simulink model "ZAD2_Model"  (R2018a)
settings: Solver=ode45  StartTime=0.0  StopTime=tend  MaxStep=Tp  RelTol=1e-3
values from neighbouring files (symbols this model uses):
  initConditionsAcc = [0 0]    [ZAD2_Init.m]
  initConditionsVel = [0 0]    [ZAD2_Init.m]
  omega = 5.0    (= 5)    [ZAD2_Init.m]
  tauM1 = 3.0    (= 3)    [ZAD2_Init.m]
  tauM2 = 4.0    (= 4)    [ZAD2_Init.m]
libraries: simulink x4
settings Model: Creator=szymon  LastModifiedBy=szymon

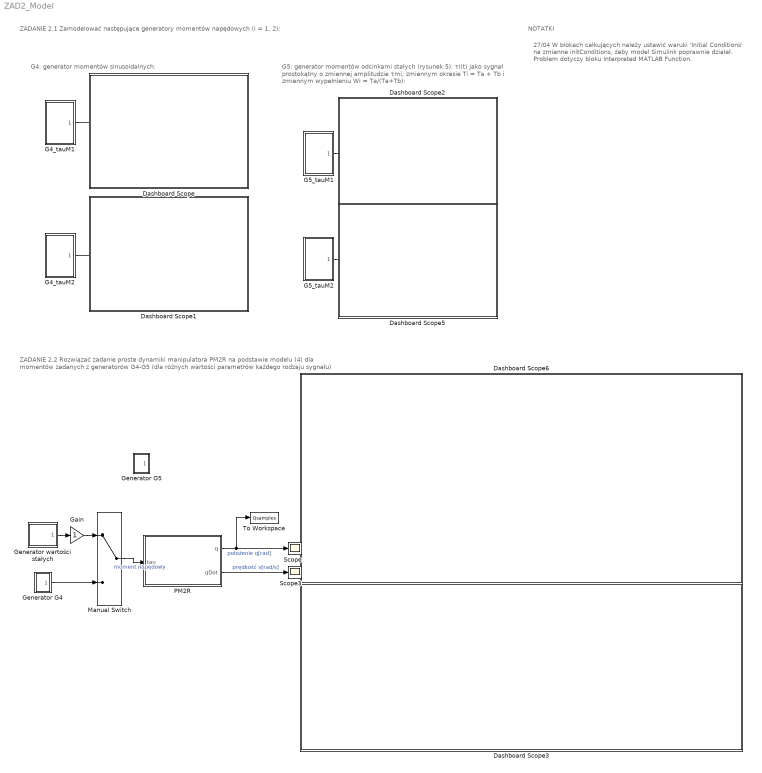
== system ZAD2_Model ==
  note: NOTATKI
  note: G4: generator momentów sinusoidalnych:
  note: ZADANIE 2.1
      | Zamodelować następujące generatory momentów napędowych (i = 1, 2):
  note: G5: generator momentów odcinkami stałych (rysunek 5):
      | τi(t) jako sygnał prostokątny o zmiennej amplitudzie τmi,
      | zmiennym okresie Ti = Ta + Tb i zmiennym wypełnieniu
      | Wi = Ta/(Ta+Tb):
  note: ZADANIE 2.2
      | Rozwiązać zadanie proste dynamiki manipulatora PM2R na podstawie modelu (4) dla momentów zadanych z generatorów G4-G5 (dla różnych wartości parametrów każdego rodzaju sygnału)
  note: 27/04 W blokach całkujących należy ustawić waruki
      | 'Initial Conditions' na zmienne initConditions, żeby model
      | Simulink poprawnie działał. Problem dotyczy bloku
      | Interpreted MATLAB Function.
  Dashboard Scope : Subsystem  DialogController=hmiCreateDDGDialog  IsWebBlock=on  mask(MWDashboardBlock){webBlockId=04488d21-9573-4550-ab8f-f6209d6c8a1b, webBlockType=sdiscope, ShowInitialText=on, HMISrcModelName=ZAD2_Model}
      mask prompts: webBlockId "WebBlock Id"; webBlockType "WebBlock Type"; HMISrcModelName "Source Model"
      mask help: SimulinkHMI:dialogs:HMIScopeDialogDesc
      mask Help: helpview([docroot '/mapfiles/simulink.map'], 'hmi_scope')
      mask Display:
      | if strcmp(get_param(bdroot(gcb),'BlockDiagramType'), 'library')
      |     image([(matlabroot) '/toolbox/simulink/hmi/icons/DashboardScope.png']);
      | end
  Dashboard Scope1 : Subsystem  DialogController=hmiCreateDDGDialog  IsWebBlock=on  mask(MWDashboardBlock){webBlockId=237970db-90af-416d-bf1d-dfbb7f9e9cad, webBlockType=sdiscope, ShowInitialText=on, HMISrcModelName=ZAD2_Model}
      mask prompts: webBlockId "WebBlock Id"; webBlockType "WebBlock Type"; HMISrcModelName "Source Model"
      mask help: SimulinkHMI:dialogs:HMIScopeDialogDesc
      mask Help: helpview([docroot '/mapfiles/simulink.map'], 'hmi_scope')
      mask Display:
      | if strcmp(get_param(bdroot(gcb),'BlockDiagramType'), 'library')
      |     image([(matlabroot) '/toolbox/simulink/hmi/icons/DashboardScope.png']);
      | end
  Dashboard Scope2 : Subsystem  DialogController=hmiCreateDDGDialog  IsWebBlock=on  mask(MWDashboardBlock){webBlockId=b7179730-6836-4ef5-be25-0ee232a07c3f, webBlockType=sdiscope, ShowInitialText=on, HMISrcModelName=ZAD2_Model}
      mask prompts: webBlockId "WebBlock Id"; webBlockType "WebBlock Type"; HMISrcModelName "Source Model"
      mask help: SimulinkHMI:dialogs:HMIScopeDialogDesc
      mask Help: helpview([docroot '/mapfiles/simulink.map'], 'hmi_scope')
      mask Display:
      | if strcmp(get_param(bdroot(gcb),'BlockDiagramType'), 'library')
      |     image([(matlabroot) '/toolbox/simulink/hmi/icons/DashboardScope.png']);
      | end
  Dashboard Scope3 : Subsystem  DialogController=hmiCreateDDGDialog  IsWebBlock=on  mask(MWDashboardBlock){webBlockId=7e31f546-b89a-4450-b53f-669fe20aafff, webBlockType=sdiscope, ShowInitialText=on, HMISrcModelName=ZAD2_Model}
      mask prompts: webBlockId "WebBlock Id"; webBlockType "WebBlock Type"; HMISrcModelName "Source Model"
      mask help: SimulinkHMI:dialogs:HMIScopeDialogDesc
      mask Help: helpview([docroot '/mapfiles/simulink.map'], 'hmi_scope')
      mask Display:
      | if strcmp(get_param(bdroot(gcb),'BlockDiagramType'), 'library')
      |     image([(matlabroot) '/toolbox/simulink/hmi/icons/DashboardScope.png']);
      | end
  Dashboard Scope5 : Subsystem  DialogController=hmiCreateDDGDialog  IsWebBlock=on  mask(MWDashboardBlock){webBlockId=43fb1c02-49ac-48a2-8cec-79fa1d2745da, webBlockType=sdiscope, ShowInitialText=on, HMISrcModelName=ZAD2_Model}
      mask prompts: webBlockId "WebBlock Id"; webBlockType "WebBlock Type"; HMISrcModelName "Source Model"
      mask help: SimulinkHMI:dialogs:HMIScopeDialogDesc
      mask Help: helpview([docroot '/mapfiles/simulink.map'], 'hmi_scope')
      mask Display:
      | if strcmp(get_param(bdroot(gcb),'BlockDiagramType'), 'library')
      |     image([(matlabroot) '/toolbox/simulink/hmi/icons/DashboardScope.png']);
      | end
  Dashboard Scope6 : Subsystem  DialogController=hmiCreateDDGDialog  IsWebBlock=on  mask(MWDashboardBlock){webBlockId=060137c1-44cd-42f9-89eb-7b1da18c6d2d, webBlockType=sdiscope, ShowInitialText=on, HMISrcModelName=ZAD2_Model}
      mask prompts: webBlockId "WebBlock Id"; webBlockType "WebBlock Type"; HMISrcModelName "Source Model"
      mask help: SimulinkHMI:dialogs:HMIScopeDialogDesc
      mask Help: helpview([docroot '/mapfiles/simulink.map'], 'hmi_scope')
      mask Display:
      | if strcmp(get_param(bdroot(gcb),'BlockDiagramType'), 'library')
      |     image([(matlabroot) '/toolbox/simulink/hmi/icons/DashboardScope.png']);
      | end
  G4_tauM1 : Subsystem
  G4_tauM2 : Subsystem
  G5_tauM1 : Subsystem
  G5_tauM2 : Subsystem
  Gain : Gain
  "Generator wartości stałych " : Subsystem
  Generator G4 : Subsystem
  Generator G5 : Subsystem
  Manual Switch : ManualSwitch
  PM2R : Subsystem
  Scope : Scope
  Scope3 : Scope
  To Workspace : ToWorkspace  VariableName=Qsamples  SampleTime=-1
  wires:
  G4_tauM1/1(G4_tauM1) -> ?
  G4_tauM2/1(G4_tauM2) -> ?
  G5_tauM2/1(G5_tauM2) -> ?
  G5_tauM1/1(G5_tauM1) -> ?
  Manual Switch/1 -> PM2R/1(tau)  "moment napędowy"
  Generator G4/1(G4) -> Manual Switch/2
  "Generator wartości stałych "/1(Gconst) -> Gain/1
  PM2R/1(q) -> To Workspace/1, Scope/1  "położenie q[rad]"
  PM2R/2(qDot) -> Scope3/1  "prędkość v[rad/s]"
  Gain/1 -> Manual Switch/1

== system ZAD2_Model/Dashboard Scope ==

== system ZAD2_Model/Dashboard Scope1 ==

== system ZAD2_Model/Dashboard Scope2 ==

== system ZAD2_Model/Dashboard Scope3 ==

== system ZAD2_Model/Dashboard Scope5 ==

== system ZAD2_Model/Dashboard Scope6 ==

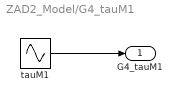
== system ZAD2_Model/G4_tauM1 ==
  "tauM1 " : Sin  Amplitude=tauM1  Frequency=omega  SampleTime=0
  G4_tauM1 : Outport
  wires:
  "tauM1 "/1 -> G4_tauM1/1

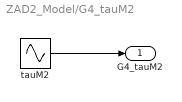
== system ZAD2_Model/G4_tauM2 ==
  "tauM2 " : Sin  Amplitude=tauM2  Frequency=omega  SampleTime=0
  G4_tauM2 : Outport
  wires:
  "tauM2 "/1 -> G4_tauM2/1

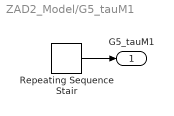
== system ZAD2_Model/G5_tauM1 ==
  Repeating Sequence Stair : simulink/Sources/Repeating Sequence Stair  OutValues=[tauM1 -tauM1 -tauM1].'  tsamp=Ta  OutMin=[]  OutMax=[]  OutDataTypeStr=double  OutputDataTypeScalingMode=double  OutDataType=fixdt(0,8)  ConRadixGroup=Best Precision: Vector-wise  OutScaling=2^-12
  G5_tauM1 : Outport
  wires:
  Repeating Sequence Stair/1 -> G5_tauM1/1

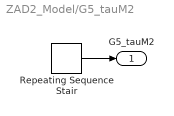
== system ZAD2_Model/G5_tauM2 ==
  Repeating Sequence Stair : simulink/Sources/Repeating Sequence Stair  OutValues=[tauM2 -tauM2 -tauM2].'  tsamp=Ta  OutMin=[]  OutMax=[]  OutDataTypeStr=double  OutputDataTypeScalingMode=double  OutDataType=fixdt(0,8)  ConRadixGroup=Best Precision: Vector-wise  OutScaling=2^-12
  G5_tauM2 : Outport
  wires:
  Repeating Sequence Stair/1 -> G5_tauM2/1

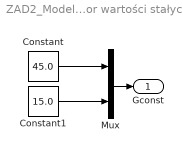
== system ZAD2_Model/Generator wartości stałych  ==
  Constant : Constant  Value=45.0
  Constant1 : Constant  Value=15.0
  Mux : Mux  Inputs=2
  Gconst : Outport
  wires:
  Constant/1 -> Mux/1
  Mux/1 -> Gconst/1
  Constant1/1 -> Mux/2

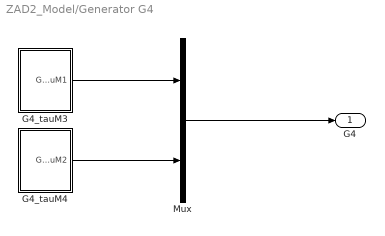
== system ZAD2_Model/Generator G4 ==
  G4_tauM3 : Subsystem
  G4_tauM4 : Subsystem
  Mux : Mux  Inputs=2
  G4 : Outport
  wires:
  G4_tauM4/1(G4_tauM2) -> Mux/2
  G4_tauM3/1(G4_tauM1) -> Mux/1
  Mux/1 -> G4/1

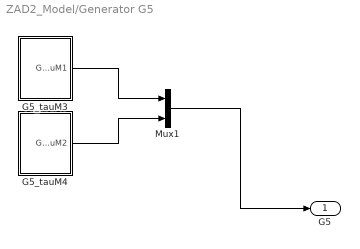
== system ZAD2_Model/Generator G5 ==
  G5_tauM3 : Subsystem
  G5_tauM4 : Subsystem
  Mux1 : Mux  Inputs=2
  G5 : Outport
  wires:
  G5_tauM4/1(G5_tauM2) -> Mux1/2
  G5_tauM3/1(G5_tauM1) -> Mux1/1
  Mux1/1 -> G5/1

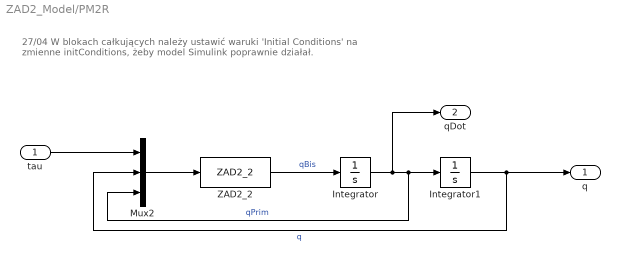
== system ZAD2_Model/PM2R ==
  note: 27/04 W blokach całkujących należy ustawić waruki 'Initial Conditions' na
      | zmienne initConditions, żeby model Simulink poprawnie działał.
  tau : Inport
  Integrator : Integrator  InitialCondition=initConditionsAcc
  Integrator1 : Integrator  InitialCondition=initConditionsVel
  Mux2 : Mux  Inputs=3
  ZAD2_2 : MATLABFcn  MATLABFcn=ZAD2_2
  q : Outport
  qDot : Outport  Port=2
  wires:
  ZAD2_2/1 -> Integrator/1  "qBis"
  Integrator/1 -> qDot/1, Mux2/3, Integrator1/1  "qPrim"
  Integrator1/1 -> q/1, Mux2/2  "q"
  tau/1 -> Mux2/1
  Mux2/1 -> ZAD2_2/1

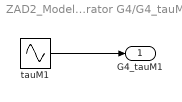
== system ZAD2_Model/Generator G4/G4_tauM3 ==
  "tauM1 " : Sin  Amplitude=tauM1  Frequency=omega  SampleTime=0
  G4_tauM1 : Outport
  wires:
  "tauM1 "/1 -> G4_tauM1/1

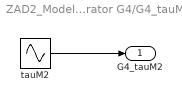
== system ZAD2_Model/Generator G4/G4_tauM4 ==
  "tauM2 " : Sin  Amplitude=tauM2  Frequency=omega  SampleTime=0
  G4_tauM2 : Outport
  wires:
  "tauM2 "/1 -> G4_tauM2/1

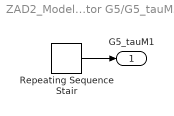
== system ZAD2_Model/Generator G5/G5_tauM3 ==
  Repeating Sequence Stair : simulink/Sources/Repeating Sequence Stair  OutValues=[tauM1 -tauM1 -tauM1].'  tsamp=Ta  OutMin=[]  OutMax=[]  OutDataTypeStr=double  OutputDataTypeScalingMode=double  OutDataType=fixdt(0,8)  ConRadixGroup=Best Precision: Vector-wise  OutScaling=2^-12
  G5_tauM1 : Outport
  wires:
  Repeating Sequence Stair/1 -> G5_tauM1/1

== system ZAD2_Model/Generator G5/G5_tauM4 ==
  Repeating Sequence Stair : simulink/Sources/Repeating Sequence Stair  OutValues=[tauM2 -tauM2 -tauM2].'  tsamp=Ta  OutMin=[]  OutMax=[]  OutDataTypeStr=double  OutputDataTypeScalingMode=double  OutDataType=fixdt(0,8)  ConRadixGroup=Best Precision: Vector-wise  OutScaling=2^-12
  G5_tauM2 : Outport
  wires:
  Repeating Sequence Stair/1 -> G5_tauM2/1
